simulink model "Manoel_06"  (R2018a)
settings: Solver=VariableStepAuto  StartTime=0.0  StopTime=30  RelTol=1e-3
values from neighbouring files (symbols this model uses):
  A = [-4.5 0; 1 -0.2]    [manoel_outubro2.m]    (also in pre6_teste.m; pre_lab5.m; pre_lab6.m; pre_pedro.m = [-5.5 0; 1 -8.40])
  B = [21.6; 0]    [manoel_outubro2.m]    (also in pre6_teste.m; pre_lab5.m = [18; 0]; pre_lab6.m = [b0; 0]; pre_pedro.m = [462; 0])
  c2_obs = [0 1]    [pre6_teste.m]    (also in pre_lab6.m)
  L1 = place(Ad',c2_obs',polos)    [pre6_teste.m]    (also in pre_lab6.m)
  L2 = place(Ad',c2_obs',[0.8998/5 + 0.2701*j 0.8998/5 - 0.2701*j])    [pre6_teste.m]    (also in pre_lab6.m = place(Ad',c2_obs',[0.8998/5 + 0.2701*i 0.8998/5 - 0.2701*i]))
  L3 = place(Ad',c2_obs',[0.92 0.82])    [pre_lab6.m]
  R0 = round(r0,1)    [naao_roda.m]    (also in pre6_teste.m; pre_lab3.m; pre_lab3_lab.m; pre_lab4.m)
  T0 = round(t0,3)    [naao_roda.m]    (also in pre6_teste.m = 0.063; pre_lab3.m; pre_lab3_2.m = 0.0640576; pre_lab3_lab.m)
undefined symbols (not defined in the file or in its folder): Ad, Bd
settings Model: Creator=joaovitor  LastModifiedBy=joaovitor

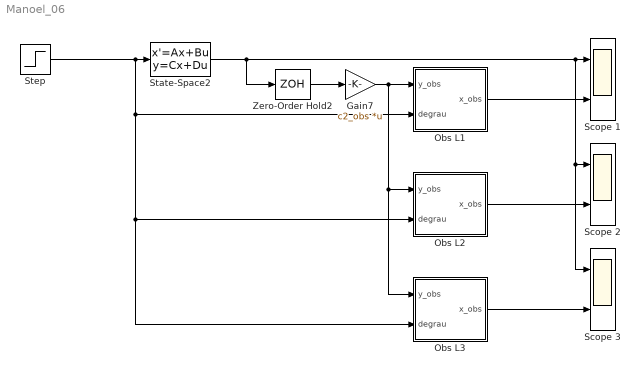
== system Manoel_06 ==
  Gain7 : Gain  Gain=c2_obs  Multiplication=Matrix(K*u)
  "Obs L1 " : MATLAB Function  TreatAsAtomicUnit=on
  Obs L2 : MATLAB Function  TreatAsAtomicUnit=on
  Obs L3 : MATLAB Function  TreatAsAtomicUnit=on
  Scope 1 : Scope  NumInputPorts=2
  Scope 2 : Scope  NumInputPorts=2
  Scope 3 : Scope  NumInputPorts=2
  State-Space2 : StateSpace  A=A  B=B  C=[1 0; 0 1]  D=[0; 0]  InitialCondition=0
  Step : Step  Time=0  After=R0  SampleTime=T0
  Zero-Order Hold2 : ZeroOrderHold  SampleTime=T0
  wires:
  Step/1 -> "Obs L1 "/2(degrau), Obs L2/2(degrau), Obs L3/2(degrau), State-Space2/1
  Zero-Order Hold2/1 -> Gain7/1
  State-Space2/1 -> Scope 1/1, Scope 3/1, Scope 2/1, Zero-Order Hold2/1
  Obs L2/1(x_obs) -> Scope 2/2
  Obs L3/1(x_obs) -> Scope 3/2
  Gain7/1 -> Obs L2/1(y_obs), Obs L3/1(y_obs), "Obs L1 "/1(y_obs)
  "Obs L1 "/1(x_obs) -> Scope 1/2

== matlab function Manoel_06/Obs L2 ==
  data: y_obs input; degrau input; Ad parameter; Bd parameter; x_obs output; L2 parameter; c2_obs parameter
function x_obs = fcn(y_obs, degrau, Ad, Bd, L2, c2_obs)

persistent x0 u0 y0
if isempty(u0)
    x0 = [12; -12];
    u0 = 0;
    y0 = 0;
end

x_obs = (Ad -L2'*c2_obs)*x0 + Bd*u0 + L2'*y0;
u0 = degrau;
y0 = y_obs;
x0 = x_obs;

== matlab function Manoel_06/Obs L1  ==
  data: y_obs input; degrau input; Ad parameter; Bd parameter; x_obs output; L1 parameter; c2_obs parameter
function x_obs = fcn(y_obs, degrau, Ad, Bd, L1, c2_obs)

persistent x0 u0 y0
if isempty(u0)
    x0 = [12; 12];
    u0 = 0;
    y0 = 0;
end

x_obs = (Ad -L1'*c2_obs)*x0 + Bd*u0 + L1'*y0;
u0 = degrau;
y0 = y_obs;
x0 = x_obs;

== matlab function Manoel_06/Obs L3 ==
  data: y_obs input; degrau input; Ad parameter; Bd parameter; x_obs output; L3 parameter; c2_obs parameter
function x_obs = fcn(y_obs, degrau, Ad, Bd, L3, c2_obs)

persistent x0 u0 y0
if isempty(u0)
    x0 = [12; -12];
    u0 = 0;
    y0 = 0;
end

x_obs = (Ad -L3'*c2_obs)*x0 + Bd*u0 + L3'*y0;
u0 = degrau;
y0 = y_obs;
x0 = x_obs;
